simulink model "design_project_closedloop_obsv_track_linear"  (R2023b)
settings: Solver=FixedStepAuto  StartTime=0.0  StopTime=20  FixedStep=0.01  RelTol=1e-3
values from neighbouring files (symbols this model uses):
  delta_x_0 = 0    [design_project.m]
  delta_y_0 = 0    [design_project.m]
  K = lqr(A, B, Q, R)*0.01    [design_project.m]
  K_i = -0.1    [design_project.m]
  L = K'    [design_project.m]
  noise = 0.0001    [design_project.m]
  r = [2; 1]    [design_project.m]
  x_0 = [1; 1; 1; 1]    [design_project.m]
libraries: simulink x1
settings Model: Creator=qingyu  LastModifiedBy=qingyu

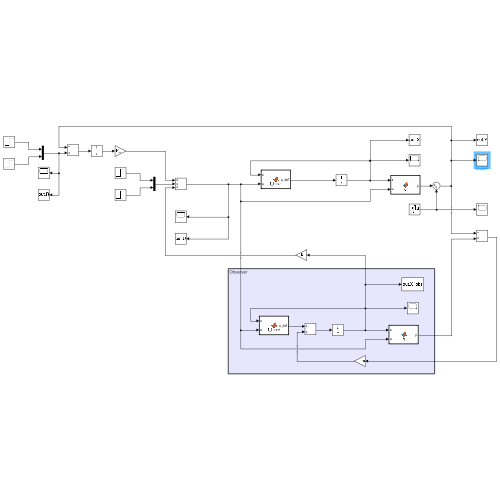
[thumbnail: Simulink's stored preview of the top-level diagram]
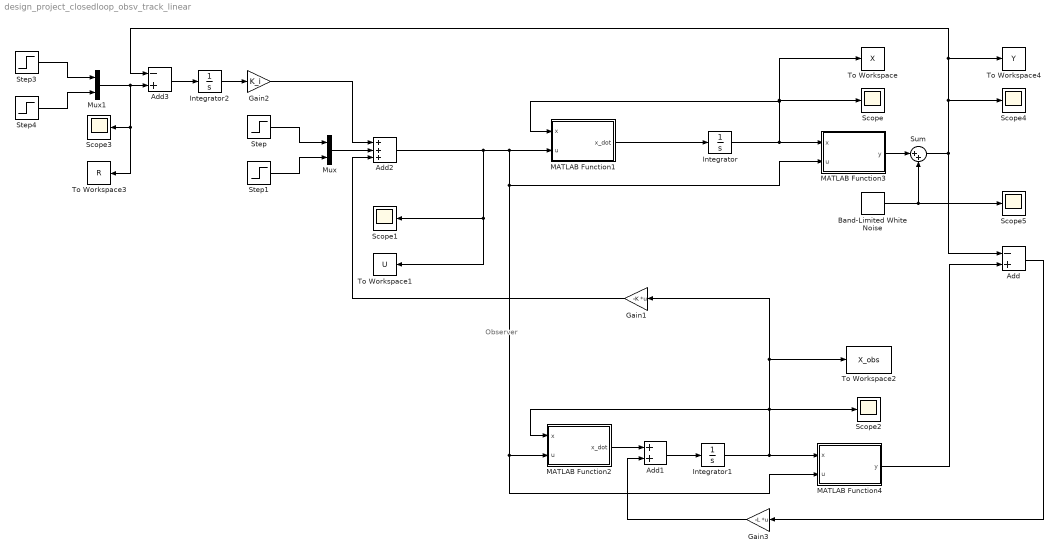
== system design_project_closedloop_obsv_track_linear ==
  note: Observer
  Add : Sum  Inputs=-+
  Add1 : Sum
  Add2 : Sum  Inputs=+++
  Add3 : Sum  Inputs=-+
  Band-Limited White Noise : simulink/Sources/Band-Limited White Noise  Cov=[noise]  Ts=0.01  seed=[23341]
  Gain1 : Gain  Gain=-K  Multiplication=Matrix(K*u)
  Gain2 : Gain  Gain=K_i
  Gain3 : Gain  Gain=-L  Multiplication=Matrix(K*u)
  Integrator : Integrator  InitialCondition=x_0
  Integrator1 : Integrator  InitialCondition=x_0
  Integrator2 : Integrator
  MATLAB Function1 : MATLAB Function  TreatAsAtomicUnit=on
  MATLAB Function2 : MATLAB Function  TreatAsAtomicUnit=on
  MATLAB Function3 : MATLAB Function  TreatAsAtomicUnit=on
  MATLAB Function4 : MATLAB Function  TreatAsAtomicUnit=on
  Mux : Mux  Inputs=2
  Mux1 : Mux  Inputs=2
  Scope{,1..5} (6 alike) : Scope
  Step : Step  After=delta_x_0  SampleTime=0
  Step1 : Step  After=delta_y_0  SampleTime=0
  Step3 : Step  Time=10  After=r(1)  SampleTime=0
  Step4 : Step  Time=5  After=r(2)  SampleTime=0
  Sum : Sum  Inputs=|++
  To Workspace : ToWorkspace  VariableName=X  SampleTime=0.01
  To Workspace1 : ToWorkspace  VariableName=U  SampleTime=0.01
  To Workspace2 : ToWorkspace  VariableName=X_obs  SampleTime=0.01
  To Workspace3 : ToWorkspace  VariableName=R  SampleTime=0.01
  To Workspace4 : ToWorkspace  VariableName=Y  SampleTime=0.01
  wires:
  MATLAB Function1/1(x_dot) -> Integrator/1
  Integrator/1 -> To Workspace/1, Scope/1, MATLAB Function1/1(x), MATLAB Function3/1(x)
  Step/1 -> Mux/1
  Step1/1 -> Mux/2
  Add2/1 -> Scope1/1, To Workspace1/1, MATLAB Function1/2(u), MATLAB Function4/2(u), MATLAB Function2/2(u), MATLAB Function3/2(u)
  MATLAB Function2/1(x_dot) -> Add1/1
  Integrator1/1 -> Scope2/1, Gain1/1, To Workspace2/1, MATLAB Function2/1(x), MATLAB Function4/1(x)
  Sum/1 -> Add3/1, To Workspace4/1, Scope4/1, Add/1
  MATLAB Function4/1(y) -> Add/2
  Add/1 -> Gain3/1
  Gain3/1 -> Add1/2
  Add1/1 -> Integrator1/1
  Mux/1 -> Add2/2
  Gain1/1 -> Add2/3
  Mux1/1 -> To Workspace3/1, Scope3/1, Add3/2
  Add3/1 -> Integrator2/1
  Gain2/1 -> Add2/1
  Step3/1 -> Mux1/1
  Step4/1 -> Mux1/2
  Integrator2/1 -> Gain2/1
  MATLAB Function3/1(y) -> Sum/1
  Band-Limited White Noise/1 -> Scope5/1, Sum/2

== matlab function design_project_closedloop_obsv_track_linear/MATLAB Function1 ==
  data: x input; x_dot output; u input
function x_dot = f_linear(x,u)

g               =  9.81;
v               =  350.3552;
m               =  320;
P               =  20000;
alpha           =  0.2618;
theta           = -0.0688;
vartheta        =  0.1930;
Z_delta_y       = -2018.0457;
Z_beta          =  13273.1810;

J_x             =  2.601;
J_y             =  751.8960;

M_x_omega_x     = -4.8379;
M_x_omega_y     = -1.7167;
M_x_beta        = -22.8888;
M_x_delta_x     = -2.5490;
M_x_delta_y     = -2.0289;

M_y_omega_x     = -15.0379;
M_y_omega_y     = -150.3792;
M_y_beta        = -2255.6880;
M_y_beta_dot    =  0;
M_y_delta_y     = -676.7064;

omega_x = x(1);
omega_y = x(2);
beta    = x(3);
gamma   = x(4);

delta_x = u(1);
delta_y = u(2);

omega_x_dot = 0;
omega_x_dot = omega_x_dot + M_x_omega_x/J_x*omega_x;
omega_x_dot = omega_x_dot + M_x_omega_y/J_x*omega_y;
omega_x_dot = omega_x_dot + M_x_beta/J_x*beta;
omega_x_dot = omega_x_dot + M_x_delta_x/J_x*delta_x;
omega_x_dot = omega_x_dot + M_x_delta_y/J_x*delta_y;

gamma_dot = 0;
gamma_dot = gamma_dot + omega_x;
gamma_dot = gamma_dot - tand(vartheta)*omega_y;

beta_dot = 0;
beta_dot = beta_dot + cosd(theta)/cosd(vartheta)*omega_y;
beta_dot = beta_dot - (P-Z_beta)/(m*v)*beta;
beta_dot = beta_dot + (g/v)*sind(theta)*beta;
beta_dot = beta_dot + (g/v)*cosd(vartheta)*gamma;
beta_dot = beta_dot + alpha*gamma_dot;
beta_dot = beta_dot + Z_delta_y/(m*v)*delta_y;

omega_y_dot = 0;
omega_y_dot = omega_y_dot + M_y_omega_x/J_y*omega_x;
omega_y_dot = omega_y_dot + M_y_omega_y/J_y*omega_y;
omega_y_dot = omega_y_dot + M_y_beta/J_y*beta;
omega_y_dot = omega_y_dot + M_y_beta_dot/J_y*beta_dot;
omega_y_dot = omega_y_dot + M_y_delta_y/J_y*delta_y;

x_dot = [
    omega_x_dot;
    omega_y_dot;
    beta_dot;
    gamma_dot
];

== matlab function design_project_closedloop_obsv_track_linear/MATLAB Function2 ==
  data: x input; x_dot output; u input
function x_dot = f_linear(x,u)

g               =  9.81;
v               =  350.3552;
m               =  320;
P               =  20000;
alpha           =  0.2618;
theta           = -0.0688;
vartheta        =  0.1930;
Z_delta_y       = -2018.0457;
Z_beta          =  13273.1810;

J_x             =  2.601;
J_y             =  751.8960;

M_x_omega_x     = -4.8379;
M_x_omega_y     = -1.7167;
M_x_beta        = -22.8888;
M_x_delta_x     = -2.5490;
M_x_delta_y     = -2.0289;

M_y_omega_x     = -15.0379;
M_y_omega_y     = -150.3792;
M_y_beta        = -2255.6880;
M_y_beta_dot    =  0;
M_y_delta_y     = -676.7064;

omega_x = x(1);
omega_y = x(2);
beta    = x(3);
gamma   = x(4);

delta_x = u(1);
delta_y = u(2);

omega_x_dot = 0;
omega_x_dot = omega_x_dot + M_x_omega_x/J_x*omega_x;
omega_x_dot = omega_x_dot + M_x_omega_y/J_x*omega_y;
omega_x_dot = omega_x_dot + M_x_beta/J_x*beta;
omega_x_dot = omega_x_dot + M_x_delta_x/J_x*delta_x;
omega_x_dot = omega_x_dot + M_x_delta_y/J_x*delta_y;

gamma_dot = 0;
gamma_dot = gamma_dot + omega_x;
gamma_dot = gamma_dot - tand(vartheta)*omega_y;

beta_dot = 0;
beta_dot = beta_dot + cosd(theta)/cosd(vartheta)*omega_y;
beta_dot = beta_dot - (P-Z_beta)/(m*v)*beta;
beta_dot = beta_dot + (g/v)*sind(theta)*beta;
beta_dot = beta_dot + (g/v)*cosd(vartheta)*gamma;
beta_dot = beta_dot + alpha*gamma_dot;
beta_dot = beta_dot + Z_delta_y/(m*v)*delta_y;

omega_y_dot = 0;
omega_y_dot = omega_y_dot + M_y_omega_x/J_y*omega_x;
omega_y_dot = omega_y_dot + M_y_omega_y/J_y*omega_y;
omega_y_dot = omega_y_dot + M_y_beta/J_y*beta;
omega_y_dot = omega_y_dot + M_y_beta_dot/J_y*beta_dot;
omega_y_dot = omega_y_dot + M_y_delta_y/J_y*delta_y;

x_dot = [
    omega_x_dot;
    omega_y_dot;
    beta_dot;
    gamma_dot
];

== matlab function design_project_closedloop_obsv_track_linear/MATLAB Function3 ==
  data: x input; y output; u input
function y = g(x,u)

omega_x = x(1);
omega_y = x(2);
beta    = x(3);
gamma   = x(4);

delta_x = u(1);
delta_y = u(2);

y_1 = omega_x;
y_2 = beta;

y = [
    y_1;
    y_2;
];

== matlab function design_project_closedloop_obsv_track_linear/MATLAB Function4 ==
  data: x input; y output; u input
function y = g(x,u)

omega_x = x(1);
omega_y = x(2);
beta    = x(3);
gamma   = x(4);

delta_x = u(1);
delta_y = u(2);

y_1 = omega_x;
y_2 = beta;

y = [
    y_1;
    y_2;
];
